simulink model "zynqRadioHWSWQPSKAD9361AD9364SL"  (R2025a)
settings: Solver=FixedStepDiscrete  StartTime=0.0  StopTime=0.5  RelTol=1e-3
PreLoadFcn:
  | setTxBurstLength = 10000;
  | txtmsg = ['Zynq radio HW/SW Co-design ÞÞÞÞ']; % Use only printable characters
  | 
  | %------------------------------------------------------------------------------------------------------
  | if ~isequal(size(txtmsg),[1 31])
  |     error('txtmsg must contain 31 characters');
  | end
  | 
  | [dataBits,msg] = zynqRadioHWSWQPSKgenHelloworldMsg(20); % generate 20 msgs for LUT
  | msgLUT = uint8(msg);
  | dataBitsLUT = dataBits(:);
  | Rsym                = 10e3;%1.92e6;
  | Config = zynqRadioHWSWQPSKTxRxParameters;
  | fs = Rsym*Config.SamplesPerSymbol;
  | word = [txtmsg newline];  % append a new line character to txtmsg
  | 
  | % The highest clock rate is 16 times the message character rate.
  | % As the message characters are fed at highest clock to FPGA
  | % repeat each character 16 times to maintain the message rate.
  | word = repelem(word.',16,1);
  | repeatTimes = ceil(setTxBurstLength/length(word));
  | inpData = complex(repmat(uint8(word),repeatTimes,1));
  | inUseTxBurstLength = length(inpData);
PostLoadFcn:
  | hScopeConfig = get_param([gcs '/HDL_QPSK/QPSK Tx Channel QPSK Rx/QPSK Rx/Frequency and Time Synchronizer/Symbol Synchronizer/No HDL/QPSK Receiver Eye Diagram'],'ScopeConfiguration');
  | hScopeConfig.OpenAtSimulationStart = false;
  | hScopeConfig.Visible = false;
  | clear hScopeConfig
InitFcn:
  | setTxBurstLength = 10000;
  | txtmsg = ['Zynq radio HW/SW Co-design ÞÞÞÞ']; % Use only printable characters
  | 
  | %------------------------------------------------------------------------------------------------------
  | if ~isequal(size(txtmsg),[1 31])
  |     error('txtmsg must contain 31 characters');
  | end
  | 
  | [dataBits,msg] = zynqRadioHWSWQPSKgenHelloworldMsg(20); % generate 20 msgs for LUT
  | msgLUT = uint8(msg);
  | dataBitsLUT = dataBits(:);
  | Rsym                = 10e3;%1.92e6;
  | Config = zynqRadioHWSWQPSKTxRxParameters;
  | fs = Rsym*Config.SamplesPerSymbol;
  | word = [txtmsg newline];  % append a new line character to txtmsg
  | 
  | % The highest clock rate is 16 times the message character rate.
  | % As the message characters are fed at highest clock to FPGA
  | % repeat each character 16 times to maintain the message rate.
  | word = repelem(word.',16,1);
  | repeatTimes = ceil(setTxBurstLength/length(word));
  | inpData = complex(repmat(uint8(word),repeatTimes,1));
  | inUseTxBurstLength = length(inpData);
  | 
  | Config.Preamble = logical(zeros(0,1))
undefined symbols (not defined in the file or in its folder): Add, dspblkCoreblockFVToolHelper, gcbh, gse_genframes, Shift
libraries: hdlsllib x144, simulink x37, dsphdlsigops2 x3, dsphdlfiltering2 x3, whdlutilities x3, dsphdlxfrm2 x2, dsphdlmathfun2 x2, commdigbbndpm3 x2, sdrzblksprivate x1
(part 5 of 6)

== system zynqRadioHWSWQPSKAD9361AD9364SL/HDL_QPSK/QPSK Tx Channel QPSK Rx/QPSK Tx/FEC Encoder/DVB-S2 LDPC Encoder/Parity RAM ==
  pwr_data : Inport
  pwr_addr : Inport  Port=2
  pwr_enb : Inport  Port=3
  prd_addr : Inport  Port=4
  AND : Logic  IconShape=distinctive  AllPortsSameDT=off  OutDataTypeStr=boolean
  ConvertToMux : MATLAB Function  TreatAsAtomicUnit=on
  ConvertToWord : MATLAB Function  TreatAsAtomicUnit=on
  Data Type Conversion{,1..3} (4 alike) : DataTypeConversion  OutDataTypeStr=fixdt(0,1,0)  SaturateOnIntegerOverflow=off  RndMeth=Floor
  Delay : Delay  DelayLength=1
  Delay1 : Delay  DelayLength=1
  Dual Port RAM System{,1..3} (4 alike) : hdlsllib/HDL RAMs/Dual Port RAM System  RAMType=Simple dual port  AsyncRead=off  WriteOutputValue=New data  RAMInitialValue=0  allowBusInputs=off  WritesHaveOutput=on  NumReads=0  NumWrites=1  SimulateUsing=Code generation  ModelRAMDelay=on  VectorAccess=Parallel
  Mux : Mux
  Relational Operator : RelationalOperator  Operator===  OutDataTypeStr=boolean  RndMeth=Simplest  InputSameDT=off
  Selector : Selector  InputPortWidth=360  IndexOptions=Index vector (dialog)  Indices=[1:90]  OutputSizes=1
  Selector1 : Selector  InputPortWidth=360  IndexOptions=Index vector (dialog)  Indices=[91:180]  OutputSizes=1
  Selector2 : Selector  InputPortWidth=360  IndexOptions=Index vector (dialog)  Indices=[181:270]  OutputSizes=1
  Selector3 : Selector  InputPortWidth=360  IndexOptions=Index vector (dialog)  Indices=[271:360]  OutputSizes=1
  Switch : Switch  Criteria=u2 > Threshold  SaturateOnIntegerOverflow=off  InputSameDT=off
  prd_data : Outport
  wires:
  ConvertToMux/2(y2) -> Mux/2
  ConvertToMux/4(y4) -> Mux/4
  Dual Port RAM System2/1 -> ConvertToMux/4(u4)
  Dual Port RAM System/1 -> ConvertToMux/1(u1)
  Dual Port RAM System1/1 -> ConvertToMux/2(u2)
  ConvertToMux/1(y1) -> Mux/1
  ConvertToMux/3(y3) -> Mux/3
  Dual Port RAM System3/1 -> ConvertToMux/3(u3)
  Mux/1 -> Switch/3
  ConvertToWord/3(y3) -> Dual Port RAM System3/1
  Data Type Conversion2/1 -> ConvertToWord/3(u3)
  ConvertToWord/1(y1) -> Dual Port RAM System/1
  ConvertToWord/4(y4) -> Dual Port RAM System2/1
  Data Type Conversion3/1 -> ConvertToWord/4(u4)
  Selector3/1 -> Data Type Conversion3/1
  Selector1/1 -> Data Type Conversion1/1
  Data Type Conversion/1 -> ConvertToWord/1(u1)
  ConvertToWord/2(y2) -> Dual Port RAM System1/1
  pwr_data/1 -> Selector/1, Selector1/1, Selector2/1, Selector3/1, Delay/1
  Selector2/1 -> Data Type Conversion2/1
  Selector/1 -> Data Type Conversion/1
  Data Type Conversion1/1 -> ConvertToWord/2(u2)
  Switch/1 -> prd_data/1
  pwr_addr/1 -> Dual Port RAM System/2, Dual Port RAM System1/2, Dual Port RAM System2/2, Dual Port RAM System3/2, Relational Operator/1
  pwr_enb/1 -> Dual Port RAM System/3, Dual Port RAM System1/3, Dual Port RAM System3/3, Dual Port RAM System2/3, Delay1/1
  prd_addr/1 -> Dual Port RAM System/4, Relational Operator/2, Dual Port RAM System1/4, Dual Port RAM System3/4, Dual Port RAM System2/4
  Delay/1 -> Switch/1
  AND/1 -> Switch/2
  Relational Operator/1 -> AND/1
  Delay1/1 -> AND/2

== system zynqRadioHWSWQPSKAD9361AD9364SL/HDL_QPSK/QPSK Tx Channel QPSK Rx/QPSK Rx/Frequency and Time Synchronizer/Coarse Frequency Compensator/Coarse Frequency Estimator/Extract Frequency ==
  datain : Inport
  validIn : Inport  Port=2
  Complex to Magnitude-Angle HDL Optimized : dsphdlmathfun2/Complex to Magnitude-Angle  NumIterationsSource=Auto  NumIterations=10  OutputFormat=Angle  AngleFormat=Normalized  ScaleOutput=on  ScalingMethod=Shift-Add  SimulateUsing=Code generation
  Delay{1..4} (4 alike) : Delay  DelayLength=1
  Gain : Gain  Gain=1/2  ParamDataTypeStr=fixdt(0,1,1)  OutDataTypeStr=Inherit: Same as input
  Unit Delay Enabled Synchronous : hdlsllib/Discrete/Unit Delay Enabled Synchronous  InitialCondition=0.0  SampleTime=-1
  normFreqOut : Outport
  wires:
  Unit Delay Enabled Synchronous/1 -> Delay2/1
  Complex to Magnitude-Angle HDL Optimized/2 -> Unit Delay Enabled Synchronous/2
  datain/1 -> Delay1/1
  Gain/1 -> Delay3/1
  Delay1/1 -> Complex to Magnitude-Angle HDL Optimized/1
  Delay2/1 -> Gain/1
  Delay3/1 -> normFreqOut/1
  validIn/1 -> Delay4/1
  Delay4/1 -> Complex to Magnitude-Angle HDL Optimized/2
  Complex to Magnitude-Angle HDL Optimized/1 -> Unit Delay Enabled Synchronous/1

== system zynqRadioHWSWQPSKAD9361AD9364SL/HDL_QPSK/QPSK Tx Channel QPSK Rx/QPSK Rx/Frequency and Time Synchronizer/Coarse Frequency Compensator/Coarse Frequency Estimator/Integrator ==
  note: store the value in the Reg before reset
  dataIn : Inport
  validIn : Inport  Port=2
  Add1 : Sum  Inputs=|++  OutDataTypeStr=Inherit: Same as first input
  Delay : Delay  DelayLength=1
  Delay1 : Delay  DelayLength=1
  Delay2 : Delay  DelayLength=1
  Integ Reg : hdlsllib/Discrete/Unit Delay Enabled Resettable Synchronous  InitialCondition=0.0  SampleTime=-1
  Reset Generator : Subsystem
  Store Reg : hdlsllib/Discrete/Unit Delay Enabled Synchronous  InitialCondition=0.0  SampleTime=-1
  IntegOut : Outport
  IntegValid : Outport  Port=2
  wires:
  Add1/1 -> Integ Reg/1
  Integ Reg/1 -> Store Reg/1, Add1/2
  validIn/1 -> Delay2/1, Reset Generator/1(validIn)
  dataIn/1 -> Delay1/1
  Delay1/1 -> Add1/1
  Delay/1 -> IntegValid/1
  Store Reg/1 -> IntegOut/1
  Reset Generator/1(reset) -> Delay/1, Store Reg/2, Integ Reg/3
  Delay2/1 -> Integ Reg/2

== system zynqRadioHWSWQPSKAD9361AD9364SL/HDL_QPSK/QPSK Tx Channel QPSK Rx/QPSK Rx/Frequency and Time Synchronizer/Phase Ambiguity Estimation and Correction/Phase Ambiguity Corrector/Reciprocal ==
  dataIn : Inport
  Compare To Constant : simulink/Logic and Bit Operations/Compare To Constant  relop=<  const=0  OutDataTypeStr=boolean
  Data Type Conversion : DataTypeConversion  OutDataTypeStr=fixdt(1,WL,0)  ConvertRealWorld=Stored Integer (SI)  SaturateOnIntegerOverflow=off  RndMeth=Floor
  Data Type Conversion1 : DataTypeConversion  OutDataTypeStr=fixdt(0,LUTAddrWL,0)  ConvertRealWorld=Stored Integer (SI)  SaturateOnIntegerOverflow=off  RndMeth=Floor
  Data Type Conversion2 : DataTypeConversion  OutDataTypeStr=fixdt(0,WL-LUTAddrWL,0)  ConvertRealWorld=Stored Integer (SI)  SaturateOnIntegerOverflow=off  RndMeth=Floor
  Delay : Delay  DelayLength=1
  Delay1 : Delay  DelayLength=1
  Delay2 : Delay  DelayLength=1
  Extract Bits : simulink/Logic and Bit Operations/Extract Bits  bitsToExtract=Range ending with least significant bit  numBits=LUTAddrWL  bitIdxRange=[0 7]  outScalingMode=Treat bit field as an integer
  Function Impl : Subsystem
  dataOut : Outport
  wires:
  dataIn/1 -> Data Type Conversion/1
  Extract Bits/1 -> Delay2/1
  Data Type Conversion/1 -> Delay/1
  Compare To Constant/1 -> Delay1/1
  Data Type Conversion1/1 -> Function Impl/2(LUTAddr)
  Function Impl/1(functionValues) -> dataOut/1
  Delay/1 -> Compare To Constant/1, Extract Bits/1
  Delay1/1 -> Data Type Conversion2/1
  Delay2/1 -> Data Type Conversion1/1
  Data Type Conversion2/1 -> Function Impl/1(switch)

== system zynqRadioHWSWQPSKAD9361AD9364SL/HDL_QPSK/QPSK Tx Channel QPSK Rx/QPSK Rx/Frequency and Time Synchronizer/Phase Ambiguity Estimation and Correction/Phase Ambiguity Estimator/Subsystem ==
  L : Inport
  H : Inport  Port=2
  Delay6 : Delay  DelayLength=1  InitialCondition=1
  Logical Operator : Logic  AllPortsSameDT=off  OutDataTypeStr=boolean
  Logical Operator1 : Logic  Operator=NOT  IconShape=distinctive  AllPortsSameDT=off  OutDataTypeStr=boolean
  Logical Operator2 : Logic  Operator=OR  AllPortsSameDT=off  OutDataTypeStr=boolean
  Out2 : Outport
  wires:
  L/1 -> Logical Operator1/1
  H/1 -> Logical Operator2/1
  Delay6/1 -> Out2/1, Logical Operator/2
  Logical Operator1/1 -> Logical Operator/1
  Logical Operator/1 -> Logical Operator2/2
  Logical Operator2/1 -> Delay6/1

== system zynqRadioHWSWQPSKAD9361AD9364SL/HDL_QPSK/QPSK Tx Channel QPSK Rx/QPSK Rx/Frequency and Time Synchronizer/Phase Ambiguity Estimation and Correction/Phase Ambiguity Estimator/Subsystem1 ==
  In1 : Inport
  validIn : Inport  Port=2
  Logical Operator1 : Logic  IconShape=distinctive  AllPortsSameDT=off  OutDataTypeStr=boolean
  Logical Operator2 : Logic  Operator=NOT  IconShape=distinctive  AllPortsSameDT=off  OutDataTypeStr=boolean
  validOut : Outport
  wires:
  In1/1 -> Logical Operator2/1
  validIn/1 -> Logical Operator1/2
  Logical Operator1/1 -> validOut/1
  Logical Operator2/1 -> Logical Operator1/1

== system zynqRadioHWSWQPSKAD9361AD9364SL/HDL_QPSK/QPSK Tx Channel QPSK Rx/QPSK Rx/Frequency and Time Synchronizer/Preamble Detector/Correlator/Magnitude Squared ==
  In1 : Inport
  Delay1 : Delay
  Delay2 : Delay
  Delay3 : Delay
  Math Function : Math  Operator=conj
  Product : Product
  Out1 : Outport
  wires:
  In1/1 -> Math Function/1, Delay2/1
  Math Function/1 -> Delay1/1
  Product/1 -> Delay3/1
  Delay2/1 -> Product/1
  Delay1/1 -> Product/2
  Delay3/1 -> Out1/1

== system zynqRadioHWSWQPSKAD9361AD9364SL/HDL_QPSK/QPSK Tx Channel QPSK Rx/QPSK Rx/Frequency and Time Synchronizer/Preamble Detector/Correlator/Magnitude Squared and Moving Sum ==
  scaled1 : Inport
  validIn : Inport  Port=2
  Add : Sum  Inputs=|+-  OutDataTypeStr=Inherit: Same as first input
  Add1 : Sum  Inputs=|++  OutDataTypeStr=Inherit: Same as first input
  Complex to Real-Imag1 : ComplexToRealImag  Output=Real
  Delay : Delay  DelayLength=13  ShowEnablePort=on
      settings: InputPortMap=u0,e6
  Delay{1..4,6,8..10,12} (9 alike) : Delay
  Delay11 : Delay  DelayLength=11
  Delay14 : Delay  DelayLength=1  ShowEnablePort=on
      settings: InputPortMap=u0,e6
  Delay5 : Delay  DelayLength=1
  Delay7 : Delay  DelayLength=1
  Gain : Gain  Gain=ThresoldGainFac  OutDataTypeStr=Inherit: Same as input
  Math Function1 : Math  Operator=conj
  Product1 : Product
  E1 : Outport
  wires:
  Add/1 -> Delay5/1
  validIn/1 -> Delay12/1
  Delay/1 -> Add/2
  Delay14/1 -> Add1/2
  Complex to Real-Imag1/1 -> Delay3/1
  Add1/1 -> Delay11/1, Delay14/1
  Delay11/1 -> E1/1
  scaled1/1 -> Delay6/1, Math Function1/1
  Math Function1/1 -> Delay1/1
  Product1/1 -> Delay2/1
  Gain/1 -> Delay4/1
  Delay6/1 -> Product1/1
  Delay1/1 -> Product1/2
  Delay2/1 -> Complex to Real-Imag1/1
  Delay3/1 -> Gain/1
  Delay4/1 -> Delay/1, Add/1
  Delay5/1 -> Add1/1
  Delay7/1 -> Delay14/2
  Delay8/1 -> Delay/2, Delay7/1
  Delay9/1 -> Delay8/1
  Delay10/1 -> Delay9/1
  Delay12/1 -> Delay10/1

== system zynqRadioHWSWQPSKAD9361AD9364SL/HDL_QPSK/QPSK Tx Channel QPSK Rx/QPSK Rx/Frequency and Time Synchronizer/Preamble Detector/Timing Adjust/No HDL ==
  note: This subsystem generates variables required for QPSKRxVerification for validation
  validIn : Inport
  timingOffset : Inport  Port=2
  syncPulse : Inport  Port=3
  Compare To Constant : simulink/Logic and Bit Operations/Compare To Constant  relop===  const=0  OutDataTypeStr=boolean
  Delay : Delay  DelayLength=4
  Delay1 : Delay  DelayLength=4
  Frame Counter : hdlsllib/Sources/HDL Counter  CountType=Free running  CountInit=0  CountStep=1  CountMax=bitsPerPacket/2 - 1  CountFromType=Initial value  CountFrom=0  CountResetPort=off  CountLoadPort=off  CountEnbPort=on  CountDirPort=off  CountHitOutputPort=off  CountDataType=Unsigned  CountWordLen=32  CountFracLen=0  CountSampTime=1
  Logical Operator : Logic  AllPortsSameDT=off  OutDataTypeStr=boolean
  No HDL : Subsystem
  No HDL1 : Subsystem
  Symbol Counter : hdlsllib/Sources/HDL Counter  CountType=Count limited  CountInit=0  CountStep=1  CountMax=bitsPerPacket/2 - 1  CountFromType=Initial value  CountFrom=0  CountResetPort=off  CountLoadPort=off  CountEnbPort=on  CountDirPort=off  CountHitOutputPort=off  CountDataType=Unsigned  CountWordLen=nextpow2(bitsPerPacket/2 - 1)  CountFracLen=0  CountSampTime=1
  Unit Delay Enabled Synchronous : hdlsllib/Discrete/Unit Delay Enabled Synchronous  InitialCondition=0.0  SampleTime=-1
  wires:
  timingOffset/1 -> Delay1/1
  validIn/1 -> Logical Operator/2, Symbol Counter/1
  Symbol Counter/1 -> Compare To Constant/1
  Logical Operator/1 -> Unit Delay Enabled Synchronous/2, Frame Counter/1
  Compare To Constant/1 -> Logical Operator/1
  Frame Counter/1 -> Unit Delay Enabled Synchronous/1
  syncPulse/1 -> Delay/1
  Unit Delay Enabled Synchronous/1 -> No HDL1/1(frameNumber)
  Delay/1 -> No HDL/Enable, No HDL1/Enable
  Delay1/1 -> No HDL/1(timingOffset)

== system zynqRadioHWSWQPSKAD9361AD9364SL/HDL_QPSK/QPSK Tx Channel QPSK Rx/QPSK Rx/Frequency and Time Synchronizer/Symbol Synchronizer/Gardner TED/GTED ==
  In1 : Inport
  Add : Sum
  Add1 : Sum  Inputs=+-
  Add2 : Sum  Inputs=+-
  Complex to Real-Imag : ComplexToRealImag
  Delay{,1..7} (8 alike) : Delay  DelayLength=1
  Delay{8..13} (6 alike) : Delay
  Product : Product
  Product1 : Product
  Out1 : Outport
  wires:
  Product/1 -> Delay10/1
  Product1/1 -> Delay13/1
  Add/1 -> Out1/1
  In1/1 -> Complex to Real-Imag/1
  Complex to Real-Imag/1 -> Add1/2, Delay/1
  Delay3/1 -> Add1/1
  Delay/1 -> Delay1/1
  Delay2/1 -> Delay3/1
  Add1/1 -> Delay9/1
  Delay1/1 -> Delay2/1, Delay8/1
  Delay5/1 -> Delay11/1, Delay6/1
  Add2/1 -> Delay12/1
  Delay6/1 -> Delay7/1
  Delay4/1 -> Delay5/1
  Delay7/1 -> Add2/1
  Complex to Real-Imag/2 -> Add2/2, Delay4/1
  Delay8/1 -> Product/1
  Delay9/1 -> Product/2
  Delay10/1 -> Add/1
  Delay11/1 -> Product1/1
  Delay12/1 -> Product1/2
  Delay13/1 -> Add/2

== system zynqRadioHWSWQPSKAD9361AD9364SL/HDL_QPSK/QPSK Tx Channel QPSK Rx/QPSK Rx/Frequency and Time Synchronizer/Symbol Synchronizer/No HDL/No HDL ==
  data : Inport
  Enable : EnablePort
  Data Type Conversion : DataTypeConversion  OutDataTypeStr=double  SaturateOnIntegerOverflow=off  RndMeth=Floor
  QPSK Receiver Constellation 1 : ConstellationDiagram  WindowPosition=[701.000000,587.000000,357.000000,388.000000,]  ScopeFrameLocation=window  SymbolsToDisplaySource=Property  SymbolsToDisplay=10000  Title=Before Symbol Synchronization  XLimits=[-1.9386 1.9401]  YLimits=[-1.9386 1.9401]  AxesLimits=[-1.9386 1.9401]  DefaultConfigurationName=comm.scopes.ConstellationDiagramBlockCfg
      settings: OpenAtSimulationStart=off
  To Workspace : ToWorkspace  VariableName=simBeforeSS  SampleTime=-1
      settings: Save2DSignal=2-D array (concatenate along first dimension)
  wires:
  Data Type Conversion/1 -> To Workspace/1, QPSK Receiver Constellation 1/1
  data/1 -> Data Type Conversion/1

== system zynqRadioHWSWQPSKAD9361AD9364SL/HDL_QPSK/QPSK Tx Channel QPSK Rx/QPSK Rx/Frequency and Time Synchronizer/Symbol Synchronizer/Rate Handle/FIFO ==
  in : Inport
  push : Inport  Port=2
  pop : Inport  Port=3
  reset : Inport  Port=4
  Delay1 : Delay  DelayLength=1
  Pop Counter : hdlsllib/Sources/HDL Counter  CountType=Count limited  CountInit=0  CountStep=1  CountMax=fifoSize -1  CountFromType=Initial value  CountFrom=0  CountResetPort=on  CountLoadPort=off  CountEnbPort=on  CountDirPort=off  CountHitOutputPort=off  CountDataType=Unsigned  CountWordLen=nextpow2(fifoSize)  CountFracLen=0  CountSampTime=1
  Push Counter : hdlsllib/Sources/HDL Counter  CountType=Count limited  CountInit=0  CountStep=1  CountMax=fifoSize -1  CountFromType=Initial value  CountFrom=0  CountResetPort=on  CountLoadPort=off  CountEnbPort=on  CountDirPort=off  CountHitOutputPort=off  CountDataType=Unsigned  CountWordLen=nextpow2(fifoSize)  CountFracLen=0  CountSampTime=1
  Simple Dual Port RAM : hdlsllib/HDL RAMs/Simple Dual Port RAM  ram_size=nextpow2(fifoSize)
  Validate Input Push Pop : Subsystem
  out : Outport
  numEntries : Outport  Port=2
  validPop : Outport  Port=3
  wires:
  Delay1/1 -> Push Counter/1, Pop Counter/1
  in/1 -> Simple Dual Port RAM/1
  reset/1 -> Validate Input Push Pop/1(rst), Delay1/1
  Validate Input Push Pop/2(valid pop) -> Pop Counter/2, validPop/1
  Validate Input Push Pop/1(valid push) -> Push Counter/2, Simple Dual Port RAM/3
  pop/1 -> Validate Input Push Pop/3(pop)
  push/1 -> Validate Input Push Pop/2(push)
  Pop Counter/1 -> Simple Dual Port RAM/4
  Push Counter/1 -> Simple Dual Port RAM/2
  Simple Dual Port RAM/1 -> out/1
  Validate Input Push Pop/3(numEntries) -> numEntries/1

== system zynqRadioHWSWQPSKAD9361AD9364SL/HDL_QPSK/QPSK Tx Channel QPSK Rx/QPSK Tx/Bit Packetizer/Data Bits FIFO/No HDL/No HDL ==
  push : Inport
  full : Inport  Port=2
  ncount : Inport  Port=3
  empty : Inport  Port=4
  pop : Inport  Port=5
  Assertion : Assertion
  Assertion1 : Assertion
  Display : Display
  Logical Operator : Logic  Operator=NAND  AllPortsSameDT=off  OutDataTypeStr=boolean
  Logical Operator1 : Logic  Operator=NAND  AllPortsSameDT=off  OutDataTypeStr=boolean
  wires:
  Logical Operator1/1 -> Assertion1/1
  ncount/1 -> Display/1
  Logical Operator/1 -> Assertion/1
  pop/1 -> Logical Operator1/2
  full/1 -> Logical Operator/2
  empty/1 -> Logical Operator1/1
  push/1 -> Logical Operator/1

== system zynqRadioHWSWQPSKAD9361AD9364SL/HDL_QPSK/QPSK Tx Channel QPSK Rx/QPSK Tx/FEC Encoder/DVB-S2 BCH Encoder/Parity Generation/Store and Retrieve Parity ==
  iwr_data : Inport  Partition=on  PartitionDimension=1  PartitionWidth=1  PartitionOffset=0
  iwr_addr : Inport  Port=2
  iwr_enb : Inport  Port=3  Partition=on  PartitionDimension=1  PartitionWidth=1  PartitionOffset=0
  ird_addr : Inport  Port=4
  For Each : ForEach  DisableCoverage=on
  parity RAM : hdlsllib/HDL RAMs/Simple Dual Port RAM  ram_size=3
  ird_data : Outport  ConcatenationDimension=1
  wires:
  ird_addr/1 -> parity RAM/4
  iwr_data/1 -> parity RAM/1
  iwr_addr/1 -> parity RAM/2
  iwr_enb/1 -> parity RAM/3
  parity RAM/1 -> ird_data/1

== system zynqRadioHWSWQPSKAD9361AD9364SL/HDL_QPSK/QPSK Tx Channel QPSK Rx/QPSK Rx/Frequency and Time Synchronizer/Coarse Frequency Compensator/Coarse Frequency Estimator/Integrator/Reset Generator ==
  validIn : Inport
  Compare To Constant : simulink/Logic and Bit Operations/Compare To Constant  relop===  const=integAvgLen  OutDataTypeStr=boolean
  Delay1 : Delay  DelayLength=1
  Delay5 : Delay  DelayLength=1
  HDL Counter : hdlsllib/Sources/HDL Counter  CountType=Count limited  CountInit=0  CountStep=1  CountMax=integAvgLen  CountFromType=Initial value  CountFrom=0  CountResetPort=off  CountLoadPort=off  CountEnbPort=on  CountDirPort=off  CountHitOutputPort=off  CountDataType=Unsigned  CountWordLen=nextpow2(integAvgLen + 1)  CountFracLen=0  CountSampTime=1
  Logical Operator : Logic  AllPortsSameDT=off  OutDataTypeStr=boolean
  reset : Outport
  wires:
  Delay1/1 -> Logical Operator/1
  Delay5/1 -> Compare To Constant/1
  Logical Operator/1 -> reset/1
  validIn/1 -> HDL Counter/1, Delay1/1
  Compare To Constant/1 -> Logical Operator/2
  HDL Counter/1 -> Delay5/1

== system zynqRadioHWSWQPSKAD9361AD9364SL/HDL_QPSK/QPSK Tx Channel QPSK Rx/QPSK Rx/Frequency and Time Synchronizer/Phase Ambiguity Estimation and Correction/Phase Ambiguity Corrector/Reciprocal/Function Impl ==
  switch : Inport
  LUTAddr : Inport  Port=2
  Delay{6..8,10,15..16} (6 alike) : Delay
  Delay9 : Delay  DelayLength=1
  LUT1 : LookupNDDirect  NumberOfTableDimensions=1  Table=LUT(:,1)  DiagnosticForOutOfRangeInput=Error
  LUT2 : LookupNDDirect  NumberOfTableDimensions=1  Table=LUT(:,2)  DiagnosticForOutOfRangeInput=Error
  Multiport Switch : MultiPortSwitch  DataPortOrder=Zero-based contiguous  Inputs=2  zeroidx=on  SaturateOnIntegerOverflow=off  InputSameDT=off
  functionValues : Outport
  wires:
  Multiport Switch/1 -> Delay9/1
  Delay6/1 -> LUT1/1
  Delay7/1 -> LUT2/1
  Delay8/1 -> Delay10/1
  switch/1 -> Delay8/1
  LUT1/1 -> Delay16/1
  LUT2/1 -> Delay15/1
  Delay9/1 -> functionValues/1
  Delay10/1 -> Multiport Switch/1
  Delay16/1 -> Multiport Switch/3
  Delay15/1 -> Multiport Switch/2
  LUTAddr/1 -> Delay6/1, Delay7/1

== system zynqRadioHWSWQPSKAD9361AD9364SL/HDL_QPSK/QPSK Tx Channel QPSK Rx/QPSK Rx/Frequency and Time Synchronizer/Preamble Detector/Timing Adjust/No HDL/No HDL ==
  timingOffset : Inport
  Enable : EnablePort
  Data Type Conversion : DataTypeConversion  OutDataTypeStr=double  SaturateOnIntegerOverflow=off  RndMeth=Floor
  To Workspace : ToWorkspace  VariableName=simTimingOffset  SampleTime=-1
      settings: Save2DSignal=2-D array (concatenate along first dimension)
  wires:
  Data Type Conversion/1 -> To Workspace/1
  timingOffset/1 -> Data Type Conversion/1

== system zynqRadioHWSWQPSKAD9361AD9364SL/HDL_QPSK/QPSK Tx Channel QPSK Rx/QPSK Rx/Frequency and Time Synchronizer/Preamble Detector/Timing Adjust/No HDL/No HDL1 ==
  frameNumber : Inport
  Enable : EnablePort
  Data Type Conversion : DataTypeConversion  OutDataTypeStr=double  SaturateOnIntegerOverflow=off  RndMeth=Floor
  To Workspace : ToWorkspace  VariableName=simSyncedPackets  SampleTime=-1
      settings: Save2DSignal=2-D array (concatenate along first dimension)
  wires:
  frameNumber/1 -> Data Type Conversion/1
  Data Type Conversion/1 -> To Workspace/1

== system zynqRadioHWSWQPSKAD9361AD9364SL/HDL_QPSK/QPSK Tx Channel QPSK Rx/QPSK Rx/Frequency and Time Synchronizer/Symbol Synchronizer/Rate Handle/FIFO/Validate Input Push Pop ==
  rst : Inport
  push : Inport  Port=2
  pop : Inport  Port=3
  Compare To Constant : hdlsllib/Logic and Bit Operations/Compare To Constant  relop===  const=0  OutDataTypeStr=boolean
  Compare To Constant1 : hdlsllib/Logic and Bit Operations/Compare To Constant  relop===  const=fifoSize  OutDataTypeStr=boolean
  Constant : Constant  Value=true  SampleTime=-1
  Constant1 : Constant  Value=false  SampleTime=-1
  Delay : Delay  DelayLength=1
  Logical Operator1 : Logic  Operator=XOR  AllPortsSameDT=off  OutDataTypeStr=boolean
  Logical Operator2 : Logic  Operator=NOT  AllPortsSameDT=off  OutDataTypeStr=boolean
  Logical Operator{3..5,7,9} (5 alike) : Logic  AllPortsSameDT=off  OutDataTypeStr=boolean
  Logical Operator6 : Logic  Operator=NOT  AllPortsSameDT=off  OutDataTypeStr=boolean
  Logical Operator8 : Logic  Operator=NOT  AllPortsSameDT=off  OutDataTypeStr=boolean
  MATLAB Function : MATLAB Function  TreatAsAtomicUnit=on  mask{initVal=0, countToVal=fifoSize}
      mask prompts: initVal "Initial value:"; countToVal "Count to value:"
  No HDL : Subsystem
  Switch : Switch  Criteria=u2 ~= 0  SaturateOnIntegerOverflow=off  InputSameDT=off
  valid push : Outport
  valid pop : Outport  Port=2
  numEntries : Outport  Port=3
  wires:
  Logical Operator9/1 -> Logical Operator1/1, valid push/1
  Logical Operator2/1 -> Logical Operator9/2
  Logical Operator5/1 -> Logical Operator4/1
  Logical Operator8/1 -> Logical Operator5/2
  push/1 -> Logical Operator5/1, Logical Operator9/1
  Logical Operator1/1 -> MATLAB Function/2(enb)
  Logical Operator6/1 -> Logical Operator7/2
  Logical Operator7/1 -> Switch/2, valid pop/1, Logical Operator8/1, Logical Operator1/2
  Compare To Constant1/1 -> Logical Operator4/2
  Constant/1 -> Switch/3
  Logical Operator4/1 -> No HDL/1(pushFullFIFO), Logical Operator2/1  "push on full FIFO"
  Logical Operator3/1 -> No HDL/2(popEmptyFIFO), Logical Operator6/1  "pop on empty FIFO"
  Constant1/1 -> Switch/1
  MATLAB Function/1(count) -> Delay/1
  Switch/1 -> MATLAB Function/3(dir)
  pop/1 -> Logical Operator3/2, Logical Operator7/1
  Compare To Constant/1 -> Logical Operator3/1
  rst/1 -> MATLAB Function/1(rst)
  Delay/1 -> Compare To Constant1/1, numEntries/1, Compare To Constant/1

== system zynqRadioHWSWQPSKAD9361AD9364SL/HDL_QPSK/QPSK Tx Channel QPSK Rx/QPSK Rx/Frequency and Time Synchronizer/Symbol Synchronizer/Rate Handle/FIFO/Validate Input Push Pop/No HDL ==
  pushFullFIFO : Inport
  popEmptyFIFO : Inport  Port=2
  Constant2 : Constant  Value=pushFullDiag  SampleTime=-1
  Constant3 : Constant  Value=popEmptyDiag  SampleTime=-1
  MATLAB Function : MATLAB Function  TreatAsAtomicUnit=on
  wires:
  Constant2/1 -> MATLAB Function/1(pushFullDiag)
  Constant3/1 -> MATLAB Function/2(popEmptyDiag)
  popEmptyFIFO/1 -> MATLAB Function/4(popEmpty)
  pushFullFIFO/1 -> MATLAB Function/3(pushFull)

== matlab function zynqRadioHWSWQPSKAD9361AD9364SL/HDL_QPSK/QPSK Tx Channel QPSK Rx/QPSK Rx/Frequency and Time Synchronizer/Symbol Synchronizer/Rate Handle/FIFO/Validate Input Push Pop/No HDL/MATLAB Function ==
  data: pushFullDiag input; popEmptyDiag input; pushFull input; popEmpty input
function pushPopDiagnostics(pushFullDiag, popEmptyDiag, pushFull, popEmpty)
%#codegen


if(pushFull)
    switch pushFullDiag
        case 2
            warning('Push signal applied on full FIFO');
        case 3
            error('Push signal applied on full FIFO');
        otherwise
    end
end

if(popEmpty)
    switch popEmptyDiag
        case 2
            warning('Pop signal applied on empty FIFO');
        case 3
            error('Pop signal applied on empty FIFO');
        otherwise
    end
end

end

== matlab function zynqRadioHWSWQPSKAD9361AD9364SL/Mock FRFT/Subsystem/frft_filter ==
  data: sigIn input; sigOut output; validIn input size=1; validOut output size=1; thresh parameter
% Function mock_frft_filter
% Use matlab FRFT implemention to filter on a frame wise basis

function [sigOut, validOut] = frft_filter( ...
                                    sigIn, validIn, ... % Ports
                                    thresh ...          % Params
                                    )
%#codegen

% Peak suppressoion
if (~validIn)
    sigOut = complex(zeros(size(sigIn)));
    validOut = false;
else 
    sig_reg = sigIn;

    stdthresh = std(sig_reg);


    % Look for area with high variance ->

    for xit = 1:length(sigIn)
        if abs(sig_reg(xit)) > thresh
            sig_reg(xit) = 0 + 0i;
        end
    end
    sigOut = sig_reg;
    validOut = true;
end



end

== matlab function zynqRadioHWSWQPSKAD9361AD9364SL/Mock FRFT/add_chirp ==
  data: sigIn input; sigOut output; validIn input boolean; chirpEn input boolean; validOut output boolean; fs parameter; T parameter; f0 parameter; f1 parameter; sir parameter
% Function add_chirp
% Combine input with chirp signal specified by mask params
% Signal is complex 12 bit integer stored within 16 bit int.
function [sigOut, validOut] = add_chirp( ...
                                sigIn, validIn, chirpEn, ... % Ports
                                fs, T, f0, f1, sir)...            % Parameters
%#codegen

% Setup registers
persistent t_reg sig_reg
if isempty(t_reg)
    % zero 
    t_reg = double(0); 
    sig_reg = complex(double(0));

end

% Pass through signal unless chirp enabled
if(~chirpEn)
    sigOut = complex(double(sigIn));
    validOut = validIn;
% Add Chirp Signal
else
    % Unless valid, just hold output value
    if (~validIn)
        sigOut = complex(double(sig_reg));
        validOut = false;
    % If valid, add chirp
    else 
        % Complex chirp
        sigOut = complex(double(add_chirp(complex(double(sigIn)),t_reg,fs, T, f0, f1, sir)));
        validOut = true;
        
        % Time update
        if (t_reg == T)
            t_reg = 0;
        else 
            t_reg = t_reg+1/fs;
        end
    end
    
end



end
% End add_chirp

== matlab function zynqRadioHWSWQPSKAD9361AD9364SL/Mock FRFT/Subsystem/frft_transform ==
  data: sigIn input; sigOut output; validIn input size=1; validOut output size=1; p input
function [sigOut, validOut] = frft_transform( ...
                                            sigIn, validIn, p ... % ports
                                            )
%#codegen
%FRFT_TRANSFORM Peak search in FRFT domain
%   1D Maximum peak search to identify optimum FRFT power
sigOut = sigIn;
validOut = validIn;

% If no valid input, only output 0.
if (~validIn)
    validOut = false;
    sigOut = zeros(size(sigIn));
    p_max = 0;

% ValidIn
else
    sig_reg = sigIn;
    sigOut = frft(sig_reg, p);
    validOut = true;
end




end
% END frft_transform

== matlab function zynqRadioHWSWQPSKAD9361AD9364SL/Mock FRFT/Subsystem/windowing ==
  data: sigIn input size=4000; sigOut output size=4000; validIn input size=1; validOut output size=1
function [sigOut, validOut] = window_sig( ...
                                            sigIn, validIn) ... % Ports % Params
%#codegen
%FRFT_TRANSFORM Peak search in FRFT domain
%   1D Maximum peak search to identify optimum FRFT power

% If no valid input, only output 0.
if (~validIn)
    validOut = false;
    sigOut = complex(squeeze(zeros(4000,1)));
% ValidIn
else

   
    window = complex(hamming(4000));
    sigOut = window.*sigIn;
    validOut = true;

end




end
% END frft_transform

== matlab function zynqRadioHWSWQPSKAD9361AD9364SL/Mock FRFT/Subsystem/rescale1 ==
  data: sigIn input size=2000; sigOut output size=2000; validIn input size=1; validOut output size=1
function [sigOut, validOut] = rescale( ...
                                    sigIn, validIn ... % Ports
                                    )
%#codegen
%RESCALE Scale output for ADC 
%   Scale output to 12bit complex int stored in 16 bit int
sigOut = sigIn;
validOut = validIn;

% If no valid input, only output 0.
if (~validIn)
    validOut = false;
    sigOut = zeros(size(sigIn));
    p_max = 0;

% ValidIn
else
    sig_reg = sigIn;
    sigOut = frft(sig_reg, p);
    validOut = true;
end




end
% END frft_transform

== matlab function zynqRadioHWSWQPSKAD9361AD9364SL/HDL_QPSK/QPSK Tx Channel QPSK Rx/QPSK Tx/Bit Packetizer/Data Bits FIFO/No HDL/MATLAB Function ==
  data: wr input; full output; rd input; ncount output; empty output; dataBitsPerPacket parameter
function [full,ncount,empty] = fcn(wr,rd,dataBitsPerPacket)
%#codegen
     
    depth = dataBitsPerPacket*2 - 1;
    persistent count;
    if isempty(count)
        count = fi(0,0,nextpow2(depth),0,hdlfimath);
    end

    empty = (count == 0);
    full = (count > depth);
    ncount = count;

    if wr
        count(:) = count + 1;
    end
    if rd
        count(:) = count - 1;
    end

end

== matlab function zynqRadioHWSWQPSKAD9361AD9364SL/HDL_QPSK/QPSK Tx Channel QPSK Rx/channel/add_chirp ==
  data: sigIn input; sigOut output; validIn input boolean; chirpEn input boolean; validOut output boolean; fs parameter; T parameter; f0 parameter; f1 parameter; sir parameter
% Function add_chirp
% Combine input with chirp signal specified by mask params
% Signal is complex 12 bit integer stored within 16 bit int.
function [sigOut, validOut] = add_chirp( ...
                                sigIn, validIn, chirpEn, ... % Ports
                                fs, T, f0, f1, sir)...            % Parameters
%#codegen

% Setup registers
persistent t_reg sig_reg
if isempty(t_reg)
    % zero 
    t_reg = double(0); 
    sig_reg = complex(double(0));

end

% Pass through signal unless chirp enabled
if(~chirpEn)
    sigOut = complex(double(sigIn));
    validOut = validIn;
% Add Chirp Signal
else
    % Unless valid, just hold output value
    if (~validIn)
        sigOut = complex(double(sig_reg));
        validOut = false;
    % If valid, add chirp
    else 
        % Complex chirp
        sigOut = complex(double(add_chirp(complex(double(sigIn)),t_reg,fs, T, f0, f1, sir)));
        validOut = true;
        
        % Time update
        if (t_reg == T)
            t_reg = 0;
        else 
            t_reg = t_reg+1/fs;
        end
    end
    
end



end
% End add_chirp

== matlab function zynqRadioHWSWQPSKAD9361AD9364SL/HDL_QPSK/QPSK Tx Channel QPSK Rx/QPSK Tx/FEC Encoder/DVB-S2 BCH Encoder/Input controller/Sample Frame type and code rate ==
  data: Enable input; inpFrameLength output; frameTypeIn input; codeRateIdxIn input; inpParityLength output; validateFrameFlag output
function [inpFrameLength,inpParityLength,validateFrameFlag] = sampFramTypeCodeRate(Enable,frameTypeIn,codeRateIdxIn)
%#codegen
%% LUT
inputNFramLenLUT = fi([16008 21408 25728 32208 38688 43040 48408 51648 53840 57472 58192 58192 58192 58192 58192 58192]-1,0,16,0);
inputSFramLenLUT = fi([ 3072  5232  6312  7032  9552 10632 11712 12432 13152 14232 14232 14232 14232 14232 14232 14232]-1,0,14,0);

inpParityNLenLUT = fi([192 192 192 192 192 160 192 192 160 128 128 128 128 128 128 128 ]-1,0,8,0);
inpParitySLenLUT = fi([168 168 168 168 168 168 168 168 168 168 168 168 168 168 168 168]-1,0,8,0);
validateFrameLUT = fi([0 1],0,1,0);

inpFrameLength=cast(0,'like',inputNFramLenLUT);
inpParityLength = cast(0,'like',inpParityNLenLUT);
validateFrameFlag = cast(0,'like',validateFrameLUT);

persistent frameLength;
if isempty(frameLength)
    frameLength=cast(0,'like',inputNFramLenLUT);
end

persistent parityLength;
if isempty(parityLength)
    parityLength=cast(0,'like',inpParityNLenLUT);
end

persistent validateFrame;
if isempty(validateFrame)
    validateFrame=cast(0,'like',validateFrameLUT);
end

%% fetch from inputFramLenLUT
if Enable
    if (~frameTypeIn && codeRateIdxIn <= 10 ) || ( frameTypeIn && codeRateIdxIn <= 9 )
        validateFrameFlag(:) = validateFrameLUT(2);
        validateFrame(:) = validateFrameFlag;
    else
        validateFrameFlag(:) = validateFrameLUT(1);
        validateFrame(:) = validateFrameFlag;
    end
    if frameTypeIn
        inpFrameLength(:)=inputSFramLenLUT(codeRateIdxIn+1);
        frameLength(:)=inputSFramLenLUT(codeRateIdxIn+1);
        inpParityLength(:)=inpParitySLenLUT(codeRateIdxIn+1);
        parityLength(:)=inpParitySLenLUT(codeRateIdxIn+1);
    else
        inpFrameLength(:)=inputNFramLenLUT(codeRateIdxIn+1);
        frameLength(:)=inputNFramLenLUT(codeRateIdxIn+1);
        inpParityLength(:)=inpParityNLenLUT(codeRateIdxIn+1);
        parityLength(:)=inpParityNLenLUT(codeRateIdxIn+1);
    end
else
    inpFrameLength(:)=frameLength;
    inpParityLength(:)=parityLength;
    validateFrameFlag(:) = validateFrame;
end
end

== matlab function zynqRadioHWSWQPSKAD9361AD9364SL/HDL_QPSK/QPSK Tx Channel QPSK Rx/QPSK Tx/Bit Packetizer/Data Bits FIFO/RAM Frame Status Indicator ==
  data: push input; out output; pop input; dataBitsPerPacket parameter
function out = fcn(push,pop,dataBitsPerPacket)

   persistent pushCount popCount frameCount;
   if isempty(pushCount)
       pushCount = fi(0,0,nextpow2(dataBitsPerPacket),0,hdlfimath);
       frameCount = fi(0,0,2,0,hdlfimath);
       popCount = fi(0,0,nextpow2(dataBitsPerPacket),0,hdlfimath);
   end
   
   if (pushCount == dataBitsPerPacket-1) && push
       frameCount(:) = frameCount + 1;
   end
   if (popCount == dataBitsPerPacket-1) && pop
       frameCount(:) = frameCount - 1;
   end

   if push
       if pushCount == dataBitsPerPacket - 1
           pushCount(:) = 0;
       else
           pushCount(:) = pushCount + 1;
       end
   end

   if pop 
       if popCount == dataBitsPerPacket - 1
           popCount(:) = 0;
       else
           popCount(:) = popCount + 1;
       end
   end

   out = frameCount;

end

== matlab function zynqRadioHWSWQPSKAD9361AD9364SL/HDL_QPSK/QPSK Tx Channel QPSK Rx/QPSK Tx/FEC Encoder/DVB-S2 BCH Encoder/Input controller/sample bus controller function ==
  data: startIn input; sampledStartIn output; endIn input; validIn input; sampledEndIn output; enbBCHEnc output; reset output
function [sampledStartIn,sampledEndIn,enbBCHEnc,reset] = sampleBusController(startIn,endIn,validIn)
%#codegen
persistent startInTempFlag;
persistent endInFlag;

if isempty(startInTempFlag)
    startInTempFlag =  fi(0,0,1,0);
end
if isempty(endInFlag)
    endInFlag =  fi(0,0,1,0);
end

if endInFlag==1
    startInTempFlag = fi(0,0,1,0);
    endInFlag = fi(0,0,1,0);
end

if startIn==1 && validIn==1 && endIn~=1
    if startInTempFlag==1
        reset = fi(1,0,1,0); %reset
    else
        reset = fi(0,0,1,0);
    end
    sampledStartIn = fi(1,0,1,0); %startSample
    startInTempFlag = fi(1,0,1,0);
else
    sampledStartIn = fi(0,0,1,0);
    reset = fi(0,0,1,0);
end

if startInTempFlag
    enbBCHEnc = fi(1,0,1,0);
else
    enbBCHEnc = fi(0,0,1,0); 
end

if startIn~=1 && endIn==1 && validIn==1 && endInFlag~=1 && startInTempFlag==1
    sampledEndIn = fi(1,0,1,0);
    endInFlag = sampledEndIn;
else
    sampledEndIn = fi(0,0,1,0);
end

== matlab function zynqRadioHWSWQPSKAD9361AD9364SL/HDL_QPSK/QPSK Tx Channel QPSK Rx/QPSK Tx/FEC Encoder/DVB-S2 BCH Encoder/Parity Generation/parity indexing ==
  data: parityVectorInp input; parityScalarOut output; parityScalarValid input; parityIndex input; parityScalarValidOut output; parityLength input
function [parityScalarOut,parityScalarValidOut] = parityIndexing(parityVectorInp,parityScalarValid,parityIndex,parityLength)
%#codegen

parityScalarOut = cast(zeros(1,1),'like',parityScalarValid);
parityScalarValidOut = cast(zeros(1,1),'like',parityScalarValid);

if parityScalarValid 
    parityScalarOut(:) = parityVectorInp(parityIndex+1);
    parityScalarValidOut(:) = parityScalarValid;
else
    parityScalarOut(:) = zeros(1,1);
    parityScalarValidOut(:) = zeros(1,1);
end

== matlab function zynqRadioHWSWQPSKAD9361AD9364SL/HDL_QPSK/QPSK Tx Channel QPSK Rx/QPSK Tx/FEC Encoder/DVB-S2 BCH Encoder/Parity Generation/update parity bits ==
  data: readInpData input; parityBitsVector output size=192; readInpValid input; ParityCalCompFlag input; parityValidVector output; parityValid output; parityLength input; reset input
function [parityBitsVector,parityValidVector,parityValid] = parityBitsUpdater(readInpData,readInpValid,ParityCalCompFlag,parityLength,reset)
%#codegen

persistent writeParData;

parityBuffLen = 192;

if isempty(writeParData) || reset
    writeParData = cast(zeros(parityBuffLen,1),'like',readInpData);
end

parityBits =  cast(zeros(parityBuffLen,1),'like',readInpData);
parityBits(:) =  writeParData;
parityBitsVector = cast(zeros(parityBuffLen,1),'like',readInpData);
parityValidVector = cast(zeros(parityBuffLen,1),'like',readInpData);
parityValid = cast(zeros(1,1),'like',readInpData);
genPoly = cast(zeros(193,1),'like',readInpData);

genPoly192 = cast([1  1   1  0  0  1  1  1  1  0  1  0  1  0  1  0  0  1  0 ...
    0  0  0  0  0  0  1  1  0  0  1  1  0  1  1  1  0  1  1 ...
    1  1  1  0  1  0  0  0  0  1  1  1  1  0  0  0  1  0  1 ...
    1  0  0  0  0  0  0  1  0  0  1  0  0  0  1  0  0  0  1 ...
    0  0  0  0  1  0  1  0  1  1  0  0  0  0  1  1  1  0  1 ...
    1  0  0  0  1  1  0  1  1  0  0  1  1  0  1  0  0  1  1 ...
    1  1  0  0  1  1  0  0  0  0  1  0  1  0  0  0  1  1  1 ...
    0  0  0  1  0  0  0  1  0  1  0  0  0  1  1  1  0  1  0 ...
    0  0  1  0  0  0  0  1  1  1  0  0  0  0  0  1  0  1  1 ...
    1  0  0  0  0  0  1  1  0  0  1  0  0  0  1  1  1  0  0 ...
    1  0  1]','like',readInpData);
genPoly168 = cast([1  0  1  0  0  1  0  1  1  0  1  0  0  0  0  0  1  0  0 ...
    1  1  0  0  0  1  0  0  0  1  0  1  1  1  1  1  0  1  0 ...
    1  1  1  1  1  0  0  1  1  1  1  1  1  1  0  0  0  1  0 ...
    1  0  0  1  0  1  0  1  0  0  1  0  1  1  0  0  0  0  0 ...
    1  0  0  1  1  1  0  0  0  1  0  1  1  1  0  0  0  1  0 ...
    0  1  0  1  1  0  0  1  1  0  1  0  0  0  1  1  0  0  1 ...
    0  0  1  1  0  1  1  0  0  1  0  1  1  0  0  0  0  1  1 ...
    0  0  1  0  1  0  1  0  1  1  1  1  1  0  1  1  0  1  1 ...
    0  1  0  0  0  1  1  0  0  0  0  0  0  0  1  0  1]','like',readInpData);
genPoly160 = cast([1  0  0  0  1  0  0  1  1  0  1  0  0  1  1  0  1  1  0 ...
    1  1  1  0  1  0  0  0  1  1  1  0  1  1  0  0  0  0  0 ...
    0  0  1  1  0  0  0  1  0  0  1  0  0  0  1  0  1  1  1 ...
    1  1  1  0  1  1  1  1  1  0  0  0  0  0  0  1  1  1  0 ...
    1  0  1  0  0  0  0  1  1  1  1  0  0  1  0  1  0  1  1 ...
    0  1  1  1  1  1  0  0  0  1  1  0  0  1  1  0  0  0  1 ...
    0  1  0  1  0  0  0  0  1  1  1  1  1  1  1  0  1  1  0 ...
    1  1  1  0  0  1  1  0  0  0  0  1  0  1  0  1  0  0  0 ...
    0  0  0  0  0  1  1  0  1]','like',readInpData);
genPoly128 = cast([1  1  0  1  0  1  0  0  0  1  1  0  0  1  1  0  1  0  0 ...
    1  1  1  1  1  0  0  1  0  0  0  0  0  1  0  1  0  1  1 ...
    1  0  1  0  1  1  0  1  1  0  0  0  1  1  1  1  1  1  1 ...
    0  0  1  1  0  0  0  1  0  1  1  1  1  0  1  1  1  1  0 ...
    1  0  0  1  1  1  1  0  0  1  0  0  1  0  0  0  1  1  1 ...
    0  1  1  1  1  1  0  1  0  1  0  1  0  0  1  0  0  1  1 ...
    1  0  0  0  0  0  0  0  1  1  1  0  0  0  1]','like',readInpData);
switch parityLength
    case 191
        genPoly(:) = genPoly192;
    case 167
        genPoly(:) = [false(192-168,1); genPoly168 ];
    case 159
        genPoly(:) = [false(192-160,1); genPoly160 ];
    case 127
        genPoly(:) = [false(192-128,1); genPoly128 ];
    otherwise
        genPoly(:) = false(193,1);
end
parityLen192 = length(genPoly192)-1;
if readInpValid
    d = xor(readInpData, parityBits(192));
    for idxPoly = parityLen192 : -1 : 2
        if idxPoly > 192-parityLength
            parityBits(idxPoly) = xor(parityBits(idxPoly-1), (genPoly(idxPoly) & d));
        else
            parityBits(idxPoly) = false;
        end
    end
    parityBits(192-parityLength) = d;
    writeParData(:) = parityBits;
else
    parityBits(:) = writeParData;
end

if ParityCalCompFlag && parityLength == 191
    parityBitsVector(:) = flip(parityBits);
    parityValidVector(:) = ones(parityBuffLen,1);
    parityValid(:) = ones(1,1);
elseif ParityCalCompFlag && parityLength == 167
    parityBitsVector(:) = [flip(parityBits((192-167):192)); false(192-168,1)];
    parityValidVector(:) = [ones(168,1) ; zeros(192-168,1)];
    parityValid(:) = ones(1,1);
elseif ParityCalCompFlag && parityLength == 159
    parityBitsVector(:) = [flip(parityBits((192-159):192)); false(192-160,1)];
    parityValidVector(:) = [ones(160,1) ; zeros(192-160,1)];
    parityValid(:) = ones(1,1);
elseif ParityCalCompFlag && parityLength == 127
    parityBitsVector(:) = [flip(parityBits((192-127):192)); false(192-128,1)];
    parityValidVector(:) = [ones(128,1) ; zeros(192-128,1)];
    parityValid(:) = ones(1,1);
else
    parityBitsVector(:) = zeros(parityBuffLen,1);
    parityValidVector(:) = zeros(parityBuffLen,1);
    parityValid(:) = zeros(1,1);
end

== matlab function zynqRadioHWSWQPSKAD9361AD9364SL/HDL_QPSK/QPSK Tx Channel QPSK Rx/QPSK Tx/FEC Encoder/DVB-S2 LDPC Encoder/Indexing ==
  data: parity output; in_data input; input output; i_index input; par_data input; p_index input
function [parity,input]  = Indexing(in_data,i_index,par_data,p_index)

input = in_data(i_index);
parity = par_data(p_index);

== matlab function zynqRadioHWSWQPSKAD9361AD9364SL/HDL_QPSK/QPSK Tx Channel QPSK Rx/QPSK Tx/FEC Encoder/DVB-S2 LDPC Encoder/Input RAM/ConvertToMux ==
  data: u1 input; y1 output; u2 input; u3 input; u4 input; y2 output; y3 output; y4 output
function [y1,y2,y3,y4] = fcn(u1,u2,u3,u4)

persistent mux1 mux2 mux3 mux4;
if isempty(mux1)
    mux1 = zeros(90,1)>0;
    mux2 = zeros(90,1)>0;
    mux3 = zeros(90,1)>0;
    mux4 = zeros(90,1)>0;
end

for i =1:90
    mux1(i) = bitget(u1,91-i);
    mux2(i) = bitget(u2,91-i);
    mux3(i) = bitget(u3,91-i);
    mux4(i) = bitget(u4,91-i);
end


y1 = mux1;
y2 = mux2;
y3 = mux3;
y4 = mux4;

== matlab function zynqRadioHWSWQPSKAD9361AD9364SL/HDL_QPSK/QPSK Tx Channel QPSK Rx/QPSK Tx/FEC Encoder/DVB-S2 LDPC Encoder/Input RAM/ConvertToWord ==
  data: u1 input; y1 output; u2 input; u3 input; u4 input; y2 output; y3 output; y4 output
function [y1,y2,y3,y4] = convertToWord(u1,u2,u3,u4)

y1 = bitconcat(u1);
y2 = bitconcat(u2);
y3 = bitconcat(u3);
y4 = bitconcat(u4);

== matlab function zynqRadioHWSWQPSKAD9361AD9364SL/HDL_QPSK/QPSK Tx Channel QPSK Rx/QPSK Tx/FEC Encoder/DVB-S2 LDPC Encoder/Parity RAM/ConvertToMux ==
  data: u1 input; y1 output; u2 input; u3 input; u4 input; y2 output; y3 output; y4 output
function [y1,y2,y3,y4] = fcn(u1,u2,u3,u4)

persistent mux1 mux2 mux3 mux4;
if isempty(mux1)
    mux1 = zeros(90,1)>0;
    mux2 = zeros(90,1)>0;
    mux3 = zeros(90,1)>0;
    mux4 = zeros(90,1)>0;
end

for i =1:90
    mux1(i) = bitget(u1,91-i);
    mux2(i) = bitget(u2,91-i);
    mux3(i) = bitget(u3,91-i);
    mux4(i) = bitget(u4,91-i);
end


y1 = mux1;
y2 = mux2;
y3 = mux3;
y4 = mux4;

== matlab function zynqRadioHWSWQPSKAD9361AD9364SL/printData/MATLAB Function ==
  data: u input
function printData(u)
%#codegen

u = bitand(u,0b01111111);

 if (u ~= 10) && ((u < 32) || (u > 192))
     u(:) = 94;  % print ^ for non printable characters except for newline 
 end
 
 fprintf('%c',char(u));
end

== matlab function zynqRadioHWSWQPSKAD9361AD9364SL/HDL_QPSK/QPSK Tx Channel QPSK Rx/QPSK Tx/FEC Encoder/DVB-S2 LDPC Encoder/Parity RAM/ConvertToWord ==
  data: u1 input; y1 output; u2 input; u3 input; u4 input; y2 output; y3 output; y4 output
function [y1,y2,y3,y4] = convertToWord(u1,u2,u3,u4)

y1 = bitconcat(u1);
y2 = bitconcat(u2);
y3 = bitconcat(u3);
y4 = bitconcat(u4);
